simulink library "Lib_EMTAT"  (R2023b)
settings: Solver=VariableStepAuto  StartTime=0.0  StopTime=10.0  RelTol=1e-3
undefined symbols (not defined in the file or in its folder): MWS
libraries: simulink x31, $bdroot x1
(part 2 of 4)

== system Lib_EMTAT/Components/Power Flow/Battery ==
  note: Sign Convention:
      | i > 0 => discharging
      | i < 0 => charging
  note: Current Demand
  note: Depth of Discharge ( $\int i dt$ )
  note: Placeholder Power Loss Calculation (P = I^2*R)
  note: 1 = Discharging
      | 0 = Charging
  note: Depth of Charge/Discharge Calculation
  note: Voltage drop across resistance
  "I, A" : Inport
  "DoD, C" : Inport  Port=2
  A*s to Ah : Gain  Gain=1/3600
  Bus Creator : BusCreator  Inputs=6
  Charge Curve (1-D Lookup Table) : Lookup_n-D  NumberOfTableDimensions=1  BreakpointsForDimension1=It_vec  Table=Vcharge_vec  ExtrapMethod=Clip  UseLastTableValue=on  InternalRulePriority=Speed  RndMeth=Simplest
  Compare To Constant : simulink/Logic and Bit Operations/Compare To Constant  relop=>=  const=0  OutDataTypeStr=boolean
  Constant : Constant  Value=ESR
  Constant1 : Constant  Value=max(It_vec)
  Discharge Curve (1-D Lookup Table) : Lookup_n-D  NumberOfTableDimensions=1  BreakpointsForDimension1=It_vec  Table=Vdischarge_vec  ExtrapMethod=Clip  UseLastTableValue=on  InternalRulePriority=Speed  RndMeth=Simplest
  Divide4 : Product  Inputs=*/
  Product5 : Product
  Product8 : Product
  Saturation : Saturate  UpperLimit=100  LowerLimit=0
  Square : Math  Operator=square
  Subtract3 : Sum  Inputs=+-
  Subtract6 : Sum  Inputs=+-
  Switch : Switch  Criteria=u2 > Threshold  SaturateOnIntegerOverflow=off  InputSameDT=off
  to % : Gain  Gain=100
  "V, V" : Outport
  Outputs : Outport  Port=2
  "Ploss, W" : Outport  Port=3
  "I, C/s " : Outport  Port=4
  wires:
  [it] -> Bus Creator/6  "DoD_C"
  A*s to Ah/1 -> [it]
  "DoD, C"/1 -> A*s to Ah/1
  to %/1 -> Saturation/1
  Compare To Constant/1 -> [State], Bus Creator/5  "State"
  [i] -> Compare To Constant/1
  Product8/1 -> "Ploss, W"/1, Bus Creator/4  "Ploss_W"
  Square/1 -> Product8/2
  Constant/1 -> [R], Product8/1
  [i] -> Square/1  "i"
  [i] -> Bus Creator/3  "I_A"
  [SoC] -> Bus Creator/2  "SoC_%"
  Divide4/1 -> to %/1
  [Vout] -> Bus Creator/1  "V_V"
  Bus Creator/1 -> Outputs/1
  "I, A"/1 -> "I, C/s "/1, [i]
  Subtract6/1 -> Divide4/1
  [it] -> Subtract6/2
  Constant1/1 -> Subtract6/1, Divide4/2
  [it] -> Charge Curve (1-D Lookup Table)/1
  Subtract3/1 -> [Vout], "V, V"/1
  [R] -> Product5/1
  [i] -> Product5/2
  Product5/1 -> Subtract3/2
  Charge Curve (1-D Lookup Table)/1 -> Switch/3
  Saturation/1 -> [SoC]
  [State] -> Switch/2
  [it] -> Discharge Curve (1-D Lookup Table)/1
  Discharge Curve (1-D Lookup Table)/1 -> Switch/1
  Switch/1 -> Subtract3/1

== system Lib_EMTAT/Components/Power Flow/Cable ==
  note: Memory block used to break algebraic loop.
  "V_1, V" : Inport
  "I, A" : Inport  Port=2
  Fail? : Inport  Port=3
  "I(t-1), A" : Inport  Port=4
  Bus Creator : BusCreator  Inputs=7
  Constant : Constant  Value=R
  Divide{,1..3} (4 alike) : Product  Inputs=**
  Failure Determination : Subsystem
  Fix Zero Voltage Problem : Subsystem
  Open Circuit Failure - Current : Subsystem
  Open Circuit Failure - Voltage : Subsystem
  Square : Math  Operator=square
  Sum : Sum  Inputs=|-+
  "V_2, V" : Outport
  Outputs : Outport  Port=2
  "Ploss, W" : Outport  Port=3
  "I, A " : Outport  Port=4
  "I(t), A" : Outport  Port=5
  wires:
  [OCFail] -> Open Circuit Failure - Voltage/1(Failed?)
  Fix Zero Voltage Problem/1(Vout) -> Open Circuit Failure - Voltage/2(Vout)
  [OCFail] -> Open Circuit Failure - Current/1(Failed?)
  Open Circuit Failure - Current/1("Iin/Iout ") -> "I, A "/1, [Iin], Divide2/2, Divide3/1, Square/1
  "I, A"/1 -> "I(t), A"/1, Open Circuit Failure - Current/2(Iin/Iout)
  Fail?/1 -> Failure Determination/1(Fail?)
  Failure Determination/1(OCFail) -> [OCFail]
  "I(t-1), A"/1 -> Divide/1
  Divide/1 -> Sum/1
  "V_1, V"/1 -> Divide2/1, Sum/2, Fix Zero Voltage Problem/2(Vin), [Vin]
  Sum/1 -> Fix Zero Voltage Problem/1("Vout "), Divide3/2
  [Iin] -> Bus Creator/3  "I_A"
  [Vout] -> Bus Creator/5  "V_2_V"
  [Vin] -> Bus Creator/4  "V_1_V"
  Bus Creator/1 -> Outputs/1
  [R] -> Bus Creator/6  "R_ohm"
  Constant/1 -> Divide1/2, [R], Divide/2
  Square/1 -> Divide1/1
  Divide1/1 -> [Ploss], "Ploss, W"/1
  [Pin] -> Bus Creator/2  "P_1_W"
  [Pout] -> Bus Creator/1  "P_2_W"
  Divide2/1 -> [Pin]
  Divide3/1 -> [Pout]
  [Ploss] -> Bus Creator/7  "Ploss_W"
  Open Circuit Failure - Voltage/1("Vout ") -> "V_2, V"/1, [Vout]

== system Lib_EMTAT/Components/Power Flow/Current Distribution ==
  "I, A" : Inport
  "Idmd, A" : Inport  Port=2
  MATLAB Function : MATLAB Function  TreatAsAtomicUnit=on
  "Isplit, A" : Outport
  wires:
  "Idmd, A"/1 -> MATLAB Function/2(Idmd)
  MATLAB Function/1(Isplit) -> "Isplit, A"/1
  "I, A"/1 -> MATLAB Function/1(I)

== system Lib_EMTAT/Components/Power Flow/Current Junction ==
  I : Inport
  MATLAB Function : MATLAB Function  TreatAsAtomicUnit=on
  Isum : Outport
  wires:
  I/1 -> MATLAB Function/1(u)
  MATLAB Function/1(y) -> Isum/1

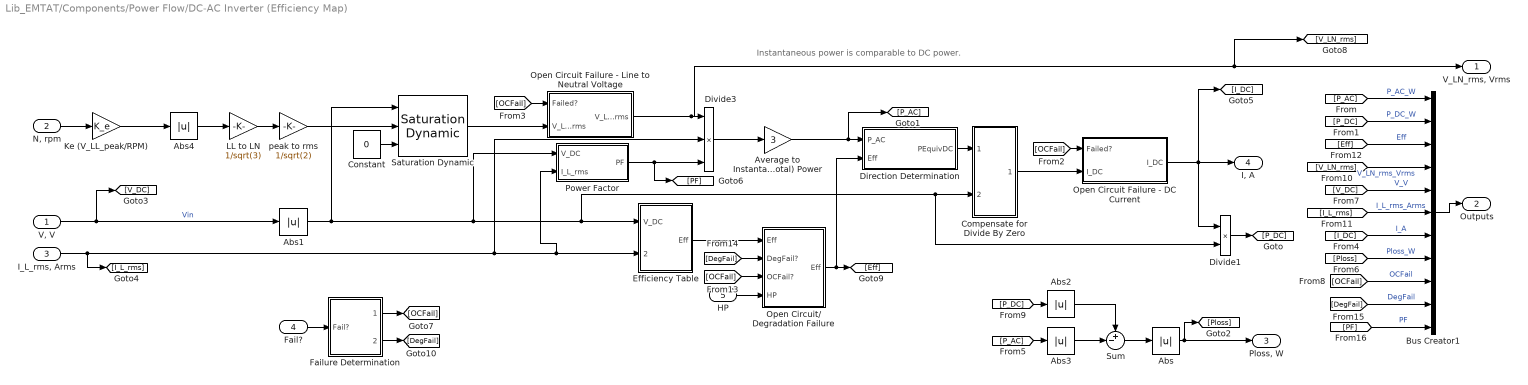
== system Lib_EMTAT/Components/Power Flow/DC-AC Inverter (Efficiency Map) ==
  note: Instantaneous power is comparable to DC power.
  "V, V" : Inport
  "N, rpm" : Inport  Port=2
  "I_L_rms, Arms" : Inport  Port=3
  Fail? : Inport  Port=4
  HP : Inport  Port=5
  Abs{,1..4} (5 alike) : Abs  SaturateOnIntegerOverflow=off
  Average to Instantaneous (Total) Power : Gain  Gain=3
  Bus Creator1 : BusCreator  Inputs=11
  Compensate for Divide By Zero : Subsystem
  Constant : Constant  Value=0
  Direction Determination : Subsystem
  Divide1 : Product  Inputs=**
  Divide3 : Product  Inputs=***
  Efficiency Table : Subsystem
  Failure Determination : Subsystem
  Ke (V_LL_peak/RPM) : Gain  Gain=K_e
  LL to LN : Gain  Gain=1/sqrt(3)
  Open Circuit Failure - DC Current : Subsystem
  Open Circuit Failure - Line to Neutral Voltage : Subsystem
  Open Circuit/ Degradation Failure : Subsystem
  Power Factor : Subsystem
  Saturation Dynamic : simulink/Discontinuities/Saturation Dynamic  OutMin=[]  OutMax=[]  OutDataTypeStr=Inherit: Same as second input  OutDataType=fixdt(1, 16)  OutScaling=2^-10  DoSatur=off
  Sum : Sum  Inputs=+-|
  peak to rms : Gain  Gain=1/sqrt(2)
  "V_LN_rms, Vrms" : Outport
  Outputs : Outport  Port=2
  "Ploss, W" : Outport  Port=3
  "I, A" : Outport  Port=4
  wires:
  peak to rms/1 -> Saturation Dynamic/2
  Constant/1 -> Saturation Dynamic/3
  Divide3/1 -> Average to Instantaneous (Total) Power/1
  Abs4/1 -> LL to LN/1
  Abs1/1 -> Power Factor/1(V_DC), Efficiency Table/1(V_DC), Compensate for Divide By Zero/2(V_DC), Divide1/2, Saturation Dynamic/1
  Divide1/1 -> [P_DC]
  Direction Determination/1(PEquivDC) -> Compensate for Divide By Zero/1(PEquivDC)
  Bus Creator1/1 -> Outputs/1
  [P_AC] -> Bus Creator1/1  "P_AC_W"
  [P_DC] -> Bus Creator1/2  "P_DC_W"
  "N, rpm"/1 -> Ke (V_LL_peak/RPM)/1
  Open Circuit/ Degradation Failure/1("Eff ") -> [Eff], Direction Determination/2(Eff)
  Open Circuit Failure - DC Current/1("I_DC ") -> Divide1/1, "I, A"/1, [I_DC]
  Average to Instantaneous (Total) Power/1 -> Direction Determination/1(P_AC), [P_AC]
  "V, V"/1 -> Abs1/1, [V_DC]  "Vin"
  Ke (V_LL_peak/RPM)/1 -> Abs4/1
  "I_L_rms, Arms"/1 -> Power Factor/2(I_L_rms), Efficiency Table/2(I_L_rms), Divide3/2, [I_L_rms]
  [V_LN_rms] -> Bus Creator1/4  "V_LN_rms_Vrms"
  [V_DC] -> Bus Creator1/5  "V_V"
  [I_DC] -> Bus Creator1/7  "I_A"
  [Ploss] -> Bus Creator1/8  "Ploss_W"
  [I_L_rms] -> Bus Creator1/6  "I_L_rms_Arms"
  [Eff] -> Bus Creator1/3  "Eff"
  LL to LN/1 -> peak to rms/1
  Compensate for Divide By Zero/1(I_DC) -> Open Circuit Failure - DC Current/2(I_DC)
  [OCFail] -> Open Circuit Failure - DC Current/1(Failed?)
  Saturation Dynamic/1 -> Open Circuit Failure - Line to Neutral Voltage/2(V_LN_rms)
  [OCFail] -> Open Circuit Failure - Line to Neutral Voltage/1(Failed?)
  Open Circuit Failure - Line to Neutral Voltage/1("V_LN_rms ") -> [V_LN_rms], "V_LN_rms, Vrms"/1, Divide3/1
  Efficiency Table/1(Eff) -> Open Circuit/ Degradation Failure/1(Eff)
  Failure Determination/2(DegFail) -> [DegFail]
  Failure Determination/1(OCFail) -> [OCFail]
  Fail?/1 -> Failure Determination/1(Fail?)
  HP/1 -> Open Circuit/ Degradation Failure/4(HP)
  [OCFail] -> Open Circuit/ Degradation Failure/3(OCFail?)
  [DegFail] -> Open Circuit/ Degradation Failure/2(DegFail?)
  Sum/1 -> Abs/1
  [P_DC] -> Abs2/1
  Abs3/1 -> Sum/2
  [P_AC] -> Abs3/1
  Abs2/1 -> Sum/1
  Abs/1 -> [Ploss], "Ploss, W"/1
  Power Factor/1(PF) -> [PF], Divide3/3
  [OCFail] -> Bus Creator1/9  "OCFail"
  [DegFail] -> Bus Creator1/10  "DegFail"
  [PF] -> Bus Creator1/11  "PF"

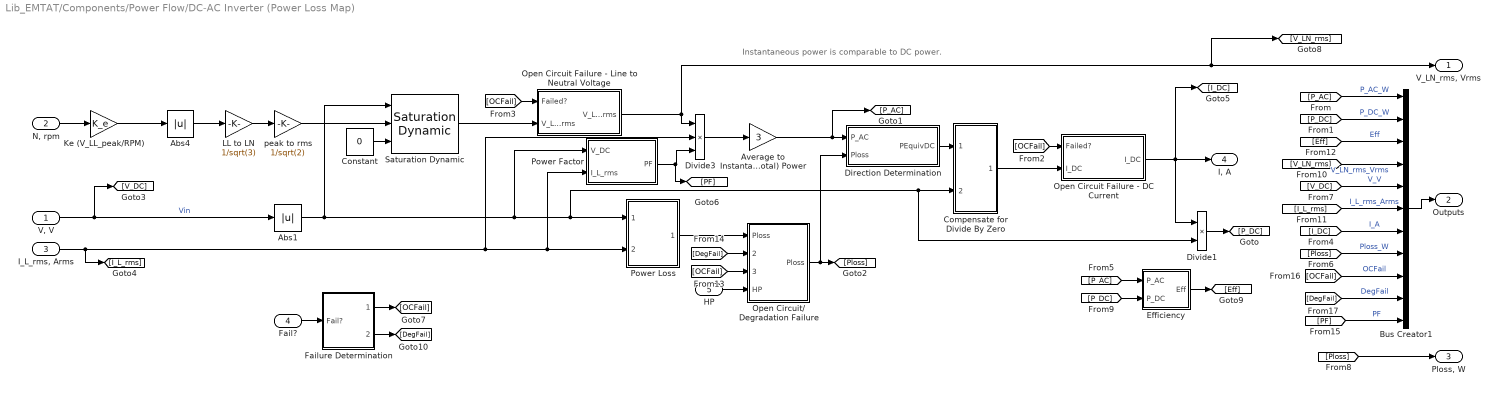
== system Lib_EMTAT/Components/Power Flow/DC-AC Inverter (Power Loss Map) ==
  note: Instantaneous power is comparable to DC power.
  "V, V" : Inport
  "N, rpm" : Inport  Port=2
  "I_L_rms, Arms" : Inport  Port=3
  Fail? : Inport  Port=4
  HP : Inport  Port=5
  Abs1 : Abs  SaturateOnIntegerOverflow=off
  Abs4 : Abs  SaturateOnIntegerOverflow=off
  Average to Instantaneous (Total) Power : Gain  Gain=3
  Bus Creator1 : BusCreator  Inputs=11
  Compensate for Divide By Zero : Subsystem
  Constant : Constant  Value=0
  Direction Determination : Subsystem
  Divide1 : Product  Inputs=**
  Divide3 : Product  Inputs=***
  Efficiency : Subsystem
  Failure Determination : Subsystem
  Ke (V_LL_peak/RPM) : Gain  Gain=K_e
  LL to LN : Gain  Gain=1/sqrt(3)
  Open Circuit Failure - DC Current : Subsystem
  Open Circuit Failure - Line to Neutral Voltage : Subsystem
  Open Circuit/ Degradation Failure : Subsystem
  Power Factor : Subsystem
  Power Loss : Subsystem
  Saturation Dynamic : simulink/Discontinuities/Saturation Dynamic  OutMin=[]  OutMax=[]  OutDataTypeStr=Inherit: Same as second input  OutDataType=fixdt(1, 16)  OutScaling=2^-10  DoSatur=off
  peak to rms : Gain  Gain=1/sqrt(2)
  "V_LN_rms, Vrms" : Outport
  Outputs : Outport  Port=2
  "Ploss, W" : Outport  Port=3
  "I, A" : Outport  Port=4
  wires:
  [DegFail] -> Open Circuit/ Degradation Failure/2(DegFail?)
  [OCFail] -> Open Circuit/ Degradation Failure/3(OCFail?)
  HP/1 -> Open Circuit/ Degradation Failure/4(HP)
  Fail?/1 -> Failure Determination/1(Fail?)
  Failure Determination/1(OCFail) -> [OCFail]
  Failure Determination/2(DegFail) -> [DegFail]
  Power Loss/1(Ploss) -> Open Circuit/ Degradation Failure/1(Ploss)
  Open Circuit Failure - Line to Neutral Voltage/1("V_LN_rms ") -> Divide3/1, "V_LN_rms, Vrms"/1, [V_LN_rms]
  [OCFail] -> Open Circuit Failure - Line to Neutral Voltage/1(Failed?)
  Saturation Dynamic/1 -> Open Circuit Failure - Line to Neutral Voltage/2(V_LN_rms)
  [OCFail] -> Open Circuit Failure - DC Current/1(Failed?)
  Compensate for Divide By Zero/1(I_DC) -> Open Circuit Failure - DC Current/2(I_DC)
  LL to LN/1 -> peak to rms/1
  [Eff] -> Bus Creator1/3  "Eff"
  Efficiency/1(Eff) -> [Eff]
  [P_AC] -> Efficiency/1(P_AC)
  [P_DC] -> Efficiency/2(P_DC)
  [I_L_rms] -> Bus Creator1/6  "I_L_rms_Arms"
  [Ploss] -> Bus Creator1/8  "Ploss_W"
  [I_DC] -> Bus Creator1/7  "I_A"
  [V_DC] -> Bus Creator1/5  "V_V"
  [V_LN_rms] -> Bus Creator1/4  "V_LN_rms_Vrms"
  "I_L_rms, Arms"/1 -> [I_L_rms], Divide3/2, Power Factor/2(I_L_rms), Power Loss/2(I_L_rms)
  [Ploss] -> "Ploss, W"/1
  Ke (V_LL_peak/RPM)/1 -> Abs4/1
  "V, V"/1 -> [V_DC], Abs1/1  "Vin"
  Average to Instantaneous (Total) Power/1 -> [P_AC], Direction Determination/1(P_AC)
  Open Circuit Failure - DC Current/1("I_DC ") -> [I_DC], "I, A"/1, Divide1/1
  Open Circuit/ Degradation Failure/1("Ploss ") -> [Ploss], Direction Determination/2(Ploss)
  "N, rpm"/1 -> Ke (V_LL_peak/RPM)/1
  [P_DC] -> Bus Creator1/2  "P_DC_W"
  [P_AC] -> Bus Creator1/1  "P_AC_W"
  Bus Creator1/1 -> Outputs/1
  Direction Determination/1(PEquivDC) -> Compensate for Divide By Zero/1(PEquivDC)
  Divide1/1 -> [P_DC]
  Abs1/1 -> Saturation Dynamic/1, Power Factor/1(V_DC), Divide1/2, Compensate for Divide By Zero/2(V_DC), Power Loss/1(V_DC)
  Abs4/1 -> LL to LN/1
  Divide3/1 -> Average to Instantaneous (Total) Power/1
  Constant/1 -> Saturation Dynamic/3
  peak to rms/1 -> Saturation Dynamic/2
  Power Factor/1(PF) -> [PF], Divide3/3
  [OCFail] -> Bus Creator1/9  "OCFail"
  [DegFail] -> Bus Creator1/10  "DegFail"
  [PF] -> Bus Creator1/11  "PF"

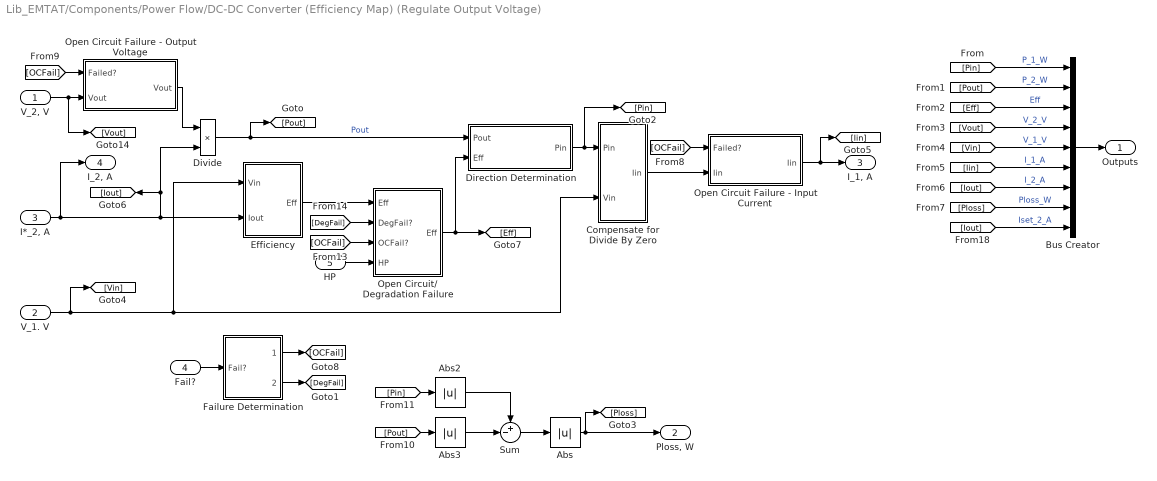
== system Lib_EMTAT/Components/Power Flow/DC-DC Converter (Efficiency Map) (Regulate Output Voltage) ==
  "V_2, V" : Inport
  V_1. V : Inport  Port=2
  "I*_2, A" : Inport  Port=3
  Fail? : Inport  Port=4
  HP : Inport  Port=5
  Abs : Abs  SaturateOnIntegerOverflow=off
  Abs2 : Abs  SaturateOnIntegerOverflow=off
  Abs3 : Abs  SaturateOnIntegerOverflow=off
  Bus Creator : BusCreator  Inputs=9
  Compensate for Divide By Zero : Subsystem
  Direction Determination : Subsystem
  Divide : Product  Inputs=**
  Efficiency : Subsystem
  Failure Determination : Subsystem
  Open Circuit Failure - Input Current : Subsystem
  Open Circuit Failure - Output Voltage : Subsystem
  Open Circuit/ Degradation Failure : Subsystem
  Sum : Sum  Inputs=+-|
  Outputs : Outport
  "Ploss, W" : Outport  Port=2
  "I_1, A" : Outport  Port=3
  "I_2, A" : Outport  Port=4
  wires:
  [Iout] -> Bus Creator/9  "Iset_2_A"
  Fail?/1 -> Failure Determination/1(Fail?)
  Failure Determination/1(OCFail) -> [OCFail]
  Failure Determination/2(DegFail) -> [DegFail]
  Efficiency/1(Eff) -> Open Circuit/ Degradation Failure/1(Eff)
  HP/1 -> Open Circuit/ Degradation Failure/4(HP)
  [DegFail] -> Open Circuit/ Degradation Failure/2(DegFail?)
  [OCFail] -> Open Circuit/ Degradation Failure/3(OCFail?)
  [OCFail] -> Open Circuit Failure - Output Voltage/1(Failed?)
  Open Circuit Failure - Output Voltage/1("Vout   ") -> Divide/1
  [OCFail] -> Open Circuit Failure - Input Current/1(Failed?)
  Compensate for Divide By Zero/1(Iin) -> Open Circuit Failure - Input Current/2(Iin)
  "V_2, V"/1 -> Open Circuit Failure - Output Voltage/2(Vout), [Vout]
  V_1. V/1 -> [Vin], Compensate for Divide By Zero/2(Vin), Efficiency/1(Vin)
  Open Circuit Failure - Input Current/1("Iin  ") -> "I_1, A"/1, [Iin]
  Open Circuit/ Degradation Failure/1("Eff ") -> Direction Determination/2(Eff), [Eff]
  Divide/1 -> Direction Determination/1(Pout), [Pout]  "Pout"
  Bus Creator/1 -> Outputs/1
  Direction Determination/1(Pin) -> [Pin], Compensate for Divide By Zero/1(Pin)
  [Pin] -> Bus Creator/1  "P_1_W"
  [Pout] -> Bus Creator/2  "P_2_W"
  [Eff] -> Bus Creator/3  "Eff"
  [Vout] -> Bus Creator/4  "V_2_V"
  [Vin] -> Bus Creator/5  "V_1_V"
  [Iin] -> Bus Creator/6  "I_1_A"
  "I*_2, A"/1 -> "I_2, A"/1, Efficiency/2(Iout), [Iout], Divide/2
  [Iout] -> Bus Creator/7  "I_2_A"
  [Pout] -> Abs3/1
  Abs3/1 -> Sum/2
  [Pin] -> Abs2/1
  Sum/1 -> Abs/1
  Abs2/1 -> Sum/1
  Abs/1 -> "Ploss, W"/1, [Ploss]
  [Ploss] -> Bus Creator/8  "Ploss_W"

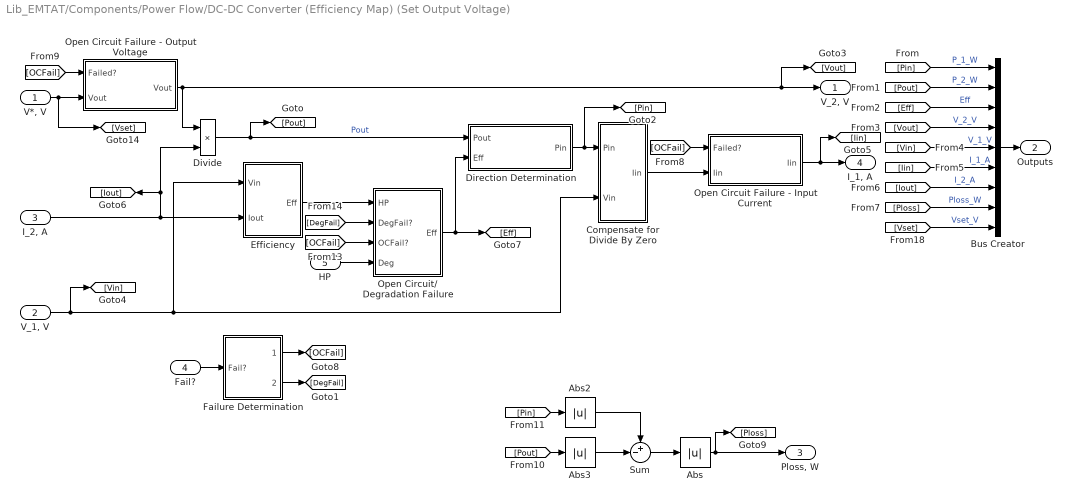
== system Lib_EMTAT/Components/Power Flow/DC-DC Converter (Efficiency Map) (Set Output Voltage) ==
  "V*, V" : Inport
  "V_1, V" : Inport  Port=2
  "I_2, A" : Inport  Port=3
  Fail? : Inport  Port=4
  HP : Inport  Port=5
  Abs : Abs  SaturateOnIntegerOverflow=off
  Abs2 : Abs  SaturateOnIntegerOverflow=off
  Abs3 : Abs  SaturateOnIntegerOverflow=off
  Bus Creator : BusCreator  Inputs=9
  Compensate for Divide By Zero : Subsystem
  Direction Determination : Subsystem
  Divide : Product  Inputs=**
  Efficiency : Subsystem
  Failure Determination : Subsystem
  Open Circuit Failure - Input Current : Subsystem
  Open Circuit Failure - Output Voltage : Subsystem
  Open Circuit/ Degradation Failure : Subsystem
  Sum : Sum  Inputs=+-|
  "V_2, V" : Outport
  Outputs : Outport  Port=2
  "Ploss, W" : Outport  Port=3
  "I_1, A" : Outport  Port=4
  wires:
  [Ploss] -> Bus Creator/8  "Ploss_W"
  [Iout] -> Bus Creator/7  "I_2_A"
  "I_2, A"/1 -> Divide/2, [Iout], Efficiency/2(Iout)
  [Iin] -> Bus Creator/6  "I_1_A"
  [Vin] -> Bus Creator/5  "V_1_V"
  [Vout] -> Bus Creator/4  "V_2_V"
  [Eff] -> Bus Creator/3  "Eff"
  [Pout] -> Bus Creator/2  "P_2_W"
  [Pin] -> Bus Creator/1  "P_1_W"
  Direction Determination/1(Pin) -> Compensate for Divide By Zero/1(Pin), [Pin]
  Bus Creator/1 -> Outputs/1
  Divide/1 -> Direction Determination/1(Pout), [Pout]  "Pout"
  Open Circuit/ Degradation Failure/1("Eff ") -> Direction Determination/2(Eff), [Eff]
  Open Circuit Failure - Input Current/1("Iin  ") -> "I_1, A"/1, [Iin]
  "V_1, V"/1 -> Efficiency/1(Vin), Compensate for Divide By Zero/2(Vin), [Vin]
  "V*, V"/1 -> [Vset], Open Circuit Failure - Output Voltage/2(Vout)
  Compensate for Divide By Zero/1(Iin) -> Open Circuit Failure - Input Current/2(Iin)
  [OCFail] -> Open Circuit Failure - Input Current/1(Failed?)
  Open Circuit Failure - Output Voltage/1("Vout   ") -> [Vout], "V_2, V"/1, Divide/1
  [OCFail] -> Open Circuit Failure - Output Voltage/1(Failed?)
  [OCFail] -> Open Circuit/ Degradation Failure/3(OCFail?)
  [DegFail] -> Open Circuit/ Degradation Failure/2(DegFail?)
  HP/1 -> Open Circuit/ Degradation Failure/4(Deg)
  Efficiency/1(Eff) -> Open Circuit/ Degradation Failure/1(HP)
  Failure Determination/2(DegFail) -> [DegFail]
  Failure Determination/1(OCFail) -> [OCFail]
  Fail?/1 -> Failure Determination/1(Fail?)
  [Vset] -> Bus Creator/9  "Vset_V"
  Abs/1 -> "Ploss, W"/1, [Ploss]
  Abs3/1 -> Sum/2
  [Pout] -> Abs3/1
  Sum/1 -> Abs/1
  Abs2/1 -> Sum/1
  [Pin] -> Abs2/1

== system Lib_EMTAT/Components/Power Flow/DC-DC Converter (Power Loss Map) (Regulate Output Voltage) ==
  "V_2, V" : Inport
  V_1. V : Inport  Port=2
  "I*_2, A" : Inport  Port=3
  Fail? : Inport  Port=4
  HP : Inport  Port=5
  Bus Creator : BusCreator  Inputs=13
  Compensate for Divide By Zero : Subsystem
  Direction Determination : Subsystem
  Divide : Product  Inputs=**
  Efficiency : Subsystem
  Failure Determination : Subsystem
  Open Circuit Failure - Input Current : Subsystem
  Open Circuit Failure - Output Voltage : Subsystem
  Open Circuit/ Degradation Failure : Subsystem
  Power Loss : Subsystem
  Outputs : Outport
  "Ploss, W" : Outport  Port=2
  "I_1, A" : Outport  Port=3
  "I_2, A" : Outport  Port=4
  wires:
  [Ploss] -> Bus Creator/8  "Ploss_W"
  [Iout] -> Bus Creator/7  "I_2_A"
  "I*_2, A"/1 -> Divide/2, [Iout], Power Loss/2(Iout), "I_2, A"/1
  [Iin] -> Bus Creator/6  "I_1_A"
  [Vin] -> Bus Creator/5  "V_1_V"
  [Vout] -> Bus Creator/4  "V_2_V"
  [Eff] -> Bus Creator/3  "Eff"
  [Pout] -> Bus Creator/2  "P_2_W"
  [Pin] -> Bus Creator/1  "P_1_W"
  Direction Determination/1(Pin) -> Compensate for Divide By Zero/1(Pin), [Pin]
  Bus Creator/1 -> Outputs/1
  Divide/1 -> Direction Determination/1(Pout), [Pout]  "Pout"
  Open Circuit/ Degradation Failure/1("Ploss ") -> "Ploss, W"/1, Direction Determination/2(Ploss), [Ploss]
  Open Circuit Failure - Input Current/1("Iin  ") -> [Iin], "I_1, A"/1
  V_1. V/1 -> Power Loss/1(Vin), Compensate for Divide By Zero/2(Vin), [Vin]
  "V_2, V"/1 -> [Vout], Open Circuit Failure - Output Voltage/2(Vout)
  [Pout] -> Efficiency/1(Pout)
  [Pin] -> Efficiency/2(Pin)
  Efficiency/1(Eff) -> [Eff]
  Compensate for Divide By Zero/1(Iin) -> Open Circuit Failure - Input Current/2(Iin)
  [OCFail] -> Open Circuit Failure - Input Current/1(Failed?)
  Open Circuit Failure - Output Voltage/1("Vout   ") -> Divide/1
  [OCFail] -> Open Circuit Failure - Output Voltage/1(Failed?)
  [OCFail] -> Open Circuit/ Degradation Failure/3(OCFail?)
  [DegFail] -> Open Circuit/ Degradation Failure/2(DegFail?)
  HP/1 -> Open Circuit/ Degradation Failure/4(HP)
  Power Loss/1(Ploss) -> Open Circuit/ Degradation Failure/1(Ploss)
  Failure Determination/2(DegFail) -> [DegFail]
  Failure Determination/1(OCFail) -> [OCFail]
  Fail?/1 -> Failure Determination/1(Fail?)
  [Iout] -> Bus Creator/9  "Iset_2_A"

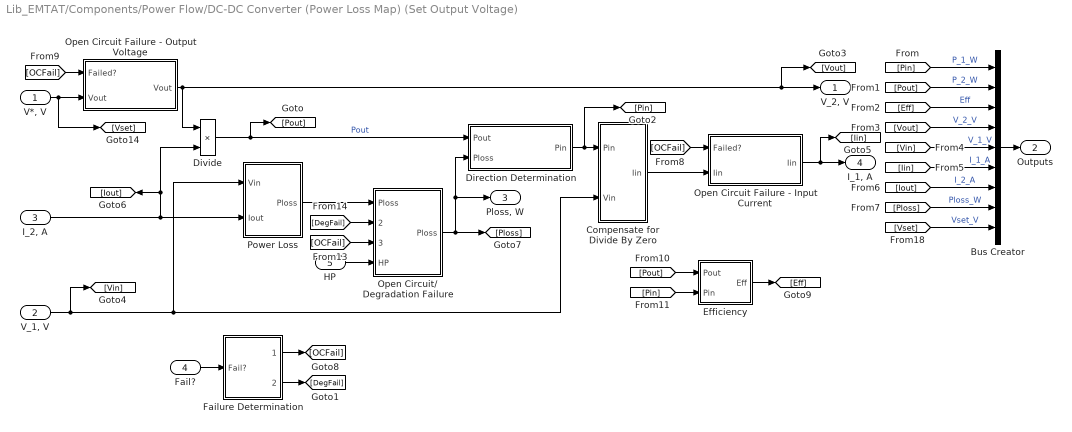
== system Lib_EMTAT/Components/Power Flow/DC-DC Converter (Power Loss Map) (Set Output Voltage) ==
  "V*, V" : Inport
  "V_1, V" : Inport  Port=2
  "I_2, A" : Inport  Port=3
  Fail? : Inport  Port=4
  HP : Inport  Port=5
  Bus Creator : BusCreator  Inputs=9
  Compensate for Divide By Zero : Subsystem
  Direction Determination : Subsystem
  Divide : Product  Inputs=**
  Efficiency : Subsystem
  Failure Determination : Subsystem
  Open Circuit Failure - Input Current : Subsystem
  Open Circuit Failure - Output Voltage : Subsystem
  Open Circuit/ Degradation Failure : Subsystem
  Power Loss : Subsystem
  "V_2, V" : Outport
  Outputs : Outport  Port=2
  "Ploss, W" : Outport  Port=3
  "I_1, A" : Outport  Port=4
  wires:
  [Vset] -> Bus Creator/9  "Vset_V"
  Fail?/1 -> Failure Determination/1(Fail?)
  Failure Determination/1(OCFail) -> [OCFail]
  Failure Determination/2(DegFail) -> [DegFail]
  Power Loss/1(Ploss) -> Open Circuit/ Degradation Failure/1(Ploss)
  HP/1 -> Open Circuit/ Degradation Failure/4(HP)
  [DegFail] -> Open Circuit/ Degradation Failure/2(DegFail?)
  [OCFail] -> Open Circuit/ Degradation Failure/3(OCFail?)
  [OCFail] -> Open Circuit Failure - Output Voltage/1(Failed?)
  Open Circuit Failure - Output Voltage/1("Vout   ") -> Divide/1, "V_2, V"/1, [Vout]
  [OCFail] -> Open Circuit Failure - Input Current/1(Failed?)
  Compensate for Divide By Zero/1(Iin) -> Open Circuit Failure - Input Current/2(Iin)
  Efficiency/1(Eff) -> [Eff]
  [Pin] -> Efficiency/2(Pin)
  [Pout] -> Efficiency/1(Pout)
  "V*, V"/1 -> Open Circuit Failure - Output Voltage/2(Vout), [Vset]
  "V_1, V"/1 -> [Vin], Compensate for Divide By Zero/2(Vin), Power Loss/1(Vin)
  Open Circuit Failure - Input Current/1("Iin  ") -> [Iin], "I_1, A"/1
  Open Circuit/ Degradation Failure/1("Ploss ") -> [Ploss], Direction Determination/2(Ploss), "Ploss, W"/1
  Divide/1 -> [Pout], Direction Determination/1(Pout)  "Pout"
  Bus Creator/1 -> Outputs/1
  Direction Determination/1(Pin) -> [Pin], Compensate for Divide By Zero/1(Pin)
  [Pin] -> Bus Creator/1  "P_1_W"
  [Pout] -> Bus Creator/2  "P_2_W"
  [Eff] -> Bus Creator/3  "Eff"
  [Vout] -> Bus Creator/4  "V_2_V"
  [Vin] -> Bus Creator/5  "V_1_V"
  [Iin] -> Bus Creator/6  "I_1_A"
  "I_2, A"/1 -> Power Loss/2(Iout), [Iout], Divide/2
  [Iout] -> Bus Creator/7  "I_2_A"
  [Ploss] -> Bus Creator/8  "Ploss_W"

== system Lib_EMTAT/Components/Power Flow/Electrical Bus ==
  "I, A" : Inport
  "V, V" : Inport  Port=2
  "Capacitance, F" : Constant  Value=C
  Divide : Product  Inputs=*/
  MATLAB Function : MATLAB Function  TreatAsAtomicUnit=on
  "V, V " : Outport
  "Vdot, V/sec" : Outport  Port=2
  wires:
  MATLAB Function/1(y) -> Divide/1
  "Capacitance, F"/1 -> Divide/2
  Divide/1 -> "Vdot, V/sec"/1
  "V, V"/1 -> "V, V "/1
  "I, A"/1 -> MATLAB Function/1(u)

== system Lib_EMTAT/Components/Power Flow/Mechanical Shaft ==
  note: Units
      | J : lb-ft-s^2
      | B : lb-ft-s
  "T, lbf-ft" : Inport
  Fail? : Inport  Port=2
  "N, rpm" : Inport  Port=3
  Abs : Abs  SaturateOnIntegerOverflow=off
  Bus Creator : BusCreator  Inputs=5
  Divide : Product  Inputs=*/
  Divide1 : Product  Inputs=**
  Failure Determination : Subsystem
  Inertia (slug-ft^2 or lbf-ft-s^2) : Constant  Value=J
  RPM to rad/s : Gain  Gain=(2*pi)/60
  Shaft Break Failure : Subsystem
  Sum : Sum  Inputs=|+-
  "Viscous Damping Coefficient, lbf-ft-s" : Gain  Gain=B
  lbf-ft to N-m : Gain  Gain=1.355818
  rad/s^2 to RPM/s : Gain  Gain=60/(2*pi)
  Outputs : Outport
  "Ploss, W" : Outport  Port=2
  "Ndot, rpm/sec" : Outport  Port=3
  wires:
  Shaft Break Failure/1("T ") -> Sum/1
  [SBFail] -> Bus Creator/5  "SBFail"
  RPM to rad/s/1 -> Divide1/2, "Viscous Damping Coefficient, lbf-ft-s"/1
  [SBFail] -> Shaft Break Failure/1(Failed?)
  Fail?/1 -> Failure Determination/1(Fail?)
  Failure Determination/1(SBFail) -> [SBFail]
  "N, rpm"/1 -> RPM to rad/s/1, [N]
  [Ndot] -> Bus Creator/3  "Ndot_rpm/sec"
  Inertia (slug-ft^2 or lbf-ft-s^2)/1 -> Divide/2
  Bus Creator/1 -> Outputs/1
  rad/s^2 to RPM/s/1 -> [Ndot], "Ndot, rpm/sec"/1
  Divide/1 -> rad/s^2 to RPM/s/1
  [Tnet] -> Bus Creator/1  "Tnet_lbf-ft"
  [N] -> Bus Creator/2  "N_rpm"
  [Ploss] -> Bus Creator/4  "Ploss_W"
  Abs/1 -> "Ploss, W"/1, [Ploss]
  Sum/1 -> [Tnet], Divide/1
  "Viscous Damping Coefficient, lbf-ft-s"/1 -> Sum/2, lbf-ft to N-m/1
  lbf-ft to N-m/1 -> Divide1/1
  "T, lbf-ft"/1 -> Shaft Break Failure/2(T)
  Divide1/1 -> Abs/1

== system Lib_EMTAT/Components/Power Flow/Power Supply (Set Voltage) ==
  "V*, V" : Inport
  "I, A" : Inport  Port=2
  Bus Creator : BusCreator  Inputs=3
  Divide : Product  Inputs=**
  MATLAB Function : MATLAB Function  TreatAsAtomicUnit=on
  Outputs : Outport
  "V, V" : Outport  Port=2
  wires:
  [Pdmd] -> Bus Creator/3  "P_W"
  [Idmdsum] -> Bus Creator/2  "Isum_A"
  [Vout] -> Bus Creator/1  "V_V"
  Divide/1 -> [Pdmd]
  Bus Creator/1 -> Outputs/1
  "V*, V"/1 -> "V, V"/1, Divide/1, [Vout]
  MATLAB Function/1(y) -> [Idmdsum], Divide/2  "Isum"
  "I, A"/1 -> MATLAB Function/1(u)

== system Lib_EMTAT/Components/Power Flow/Resistive Load Bank ==
  "V, V" : Inport
  "P*, W " : Inport  Port=2
  Fail? : Inport  Port=3
  Abs1 : Abs  SaturateOnIntegerOverflow=off
  Bus Creator : BusCreator  Inputs=5
  Divide2 : Product  Inputs=**
  Failure Determination : Subsystem
  Fix Divide By Zero. : Subsystem
  Fix Divide By Zero.1 : Subsystem
  Open Circuit Failure - Line to Neutral Voltage : Subsystem
  Square : Math  Operator=square
  Outputs : Outport
  "Ploss, W" : Outport  Port=2
  "I, A" : Outport  Port=3
  wires:
  Fix Divide By Zero.1/1(I) -> Open Circuit Failure - Line to Neutral Voltage/2(I)
  [OCFail] -> Open Circuit Failure - Line to Neutral Voltage/1(Failed?)
  Fail?/1 -> Failure Determination/1(Fail?)
  Failure Determination/1(OCFail) -> [OCFail]
  Abs1/1 -> Fix Divide By Zero./2(abs(Pset))
  Fix Divide By Zero./1(R) -> [R], Divide2/2
  Bus Creator/1 -> Outputs/1
  Square/1 -> Divide2/1, Fix Divide By Zero./1(I^2)
  "P*, W "/1 -> [Pset], Abs1/1, Fix Divide By Zero.1/2(Pset)  "Pset"
  "V, V"/1 -> [V], Fix Divide By Zero.1/1(V)  "V"
  Divide2/1 -> [Ploss], "Ploss, W"/1
  [V] -> Bus Creator/1  "V_V"
  [I] -> Bus Creator/2  "I_A"
  [Pset] -> Bus Creator/3  "Pset_W"
  [R] -> Bus Creator/4  "R_ohm"
  [Ploss] -> Bus Creator/5  "Ploss_W"
  Open Circuit Failure - Line to Neutral Voltage/1("I ") -> Square/1, [I], "I, A"/1

== system Lib_EMTAT/Components/Power Flow/Supercapacitor ==
  note: Explanation for Convention Correction:
      | If Iout is positive, discharge the capacitor. This is because a positive current demand from a sink block means that the sink block needs current.
      | If Iout is negative, charge the capacitor. This is because a negative current demand from a sink block means that the sink block is giving current.
  "I, A " : Inport
  "V, V" : Inport  Port=2
  "I(t-1), A" : Inport  Port=3
  Bus Creator : BusCreator  Inputs=5
  Constant : Constant  Value=ESR
  Convention Correction : Gain  Gain=-1
  Divide : Product  Inputs=**
  Divide1 : Product  Inputs=**
  Gain : Gain  Gain=1/C
  SOC : Subsystem
  Saturation : Saturate  UpperLimit=inf  LowerLimit=0
  Square1 : Math  Operator=square
  Sum : Sum  Inputs=|-+
  "Voltage, V to Energy, Wh" : Subsystem
  Warnings : Subsystem
  "Vout, V" : Outport
  Outputs : Outport  Port=2
  "Ploss, W" : Outport  Port=3
  "Vdot, V/sec" : Outport  Port=4
  "I(t), A" : Outport  Port=5
  wires:
  Saturation/1 -> "Voltage, V to Energy, Wh"/1(V), "Vout, V"/1, [Vout]
  "I(t-1), A"/1 -> Convention Correction/1, Divide/1
  "V, V"/1 -> Sum/2
  Divide/1 -> Sum/1
  Constant/1 -> Divide/2, Divide1/2
  Sum/1 -> Saturation/1
  [SOC] -> Warnings/1(SOC)
  "Voltage, V to Energy, Wh"/1(E) -> [Energy], SOC/1(Energy (W-h))
  "I, A "/1 -> [Iout], "I(t), A"/1
  SOC/1(SOC) -> [SOC]
  [SOC] -> Bus Creator/4  "SoC_perc"
  Divide1/1 -> [Ploss], "Ploss, W"/1
  [Ploss] -> Bus Creator/5  "Ploss_W"
  Square1/1 -> Divide1/1
  Bus Creator/1 -> Outputs/1
  [Vout] -> Bus Creator/3  "Vout_V"
  [Iout] -> Bus Creator/2  "I_A"
  [Energy] -> Bus Creator/1  "E_Wh"
  Gain/1 -> "Vdot, V/sec"/1  "Vdot"
  Convention Correction/1 -> Gain/1, Square1/1

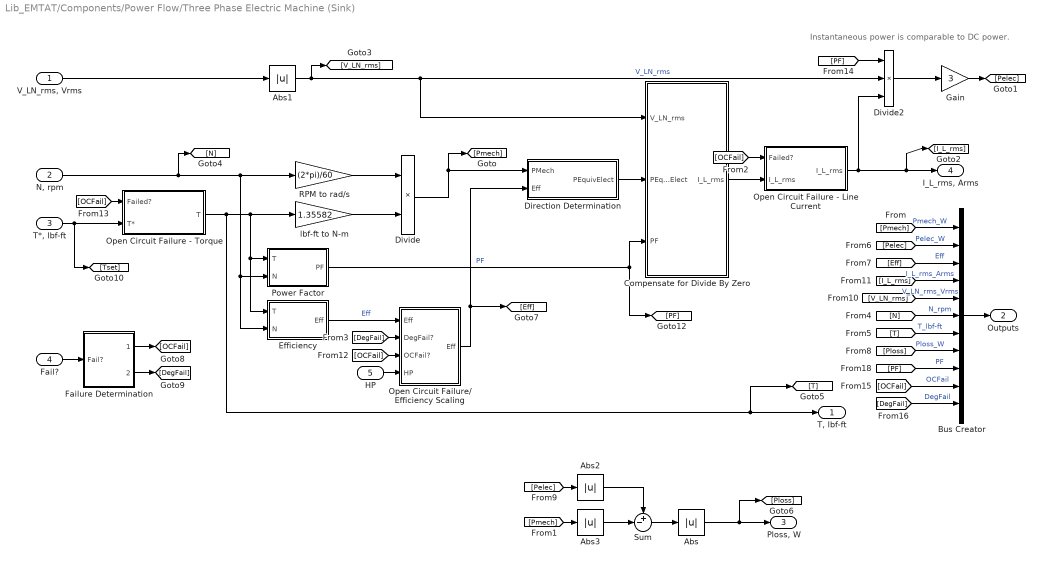
== system Lib_EMTAT/Components/Power Flow/Three Phase Electric Machine (Sink) ==
  note: Instantaneous power is comparable to DC power.
  "V_LN_rms, Vrms" : Inport
  "N, rpm" : Inport  Port=2
  "T*, lbf-ft" : Inport  Port=3
  Fail? : Inport  Port=4
  HP : Inport  Port=5
  Abs{,1..3} (4 alike) : Abs  SaturateOnIntegerOverflow=off
  Bus Creator : BusCreator  Inputs=11
  Compensate for Divide By Zero : Subsystem
  Direction Determination : Subsystem
  Divide : Product  Inputs=**
  Divide2 : Product  Inputs=***
  Efficiency : Subsystem
  Failure Determination : Subsystem
  Gain : Gain  Gain=3
  Open Circuit Failure - Line Current : Subsystem
  Open Circuit Failure - Torque : Subsystem
  Open Circuit Failure/ Efficiency Scaling : Subsystem
  Power Factor : Subsystem
  RPM to rad/s : Gain  Gain=(2*pi)/60
  Sum : Sum  Inputs=+-|
  lbf-ft to N-m : Gain  Gain=1.35582
  "T, lbf-ft" : Outport
  Outputs : Outport  Port=2
  "Ploss, W" : Outport  Port=3
  "I_L_rms, Arms" : Outport  Port=4
  wires:
  [DegFail] -> Bus Creator/11  "DegFail"
  [OCFail] -> Bus Creator/10  "OCFail"
  "T*, lbf-ft"/1 -> [Tset], Open Circuit Failure - Torque/2(T*)
  [OCFail] -> Open Circuit Failure - Torque/1(Failed?)
  [OCFail] -> Open Circuit Failure/ Efficiency Scaling/3(OCFail?)
  Fail?/1 -> Failure Determination/1(Fail?)
  HP/1 -> Open Circuit Failure/ Efficiency Scaling/4(HP)
  [DegFail] -> Open Circuit Failure/ Efficiency Scaling/2(DegFail?)
  Open Circuit Failure/ Efficiency Scaling/1("Eff ") -> [Eff], Direction Determination/2(Eff)
  Failure Determination/2(DegFail) -> [DegFail]
  Failure Determination/1(OCFail) -> [OCFail]
  [OCFail] -> Open Circuit Failure - Line Current/1(Failed?)
  Compensate for Divide By Zero/1(I_L_rms) -> Open Circuit Failure - Line Current/2(I_L_rms)
  Open Circuit Failure - Line Current/1("I_L_rms ") -> Divide2/3, "I_L_rms, Arms"/1, [I_L_rms]
  [N] -> Bus Creator/6  "N_rpm"
  [I_L_rms] -> Bus Creator/4  "I_L_rms_Arms"
  [V_LN_rms] -> Bus Creator/5  "V_LN_rms_Vrms"
  Abs1/1 -> [V_LN_rms], Compensate for Divide By Zero/1(V_LN_rms), Divide2/2  "V_LN_rms"
  Abs3/1 -> Sum/2
  [Pmech] -> Abs3/1
  Abs2/1 -> Sum/1
  [Pelec] -> Abs2/1
  Bus Creator/1 -> Outputs/1
  Efficiency/1(Eff) -> Open Circuit Failure/ Efficiency Scaling/1(Eff)  "Eff"
  "V_LN_rms, Vrms"/1 -> Abs1/1
  lbf-ft to N-m/1 -> Divide/2
  RPM to rad/s/1 -> Divide/1
  Open Circuit Failure - Torque/1("T  ") -> Power Factor/1(T), Efficiency/1(T), lbf-ft to N-m/1, "T, lbf-ft"/1, [T]
  Divide/1 -> [Pmech], Direction Determination/1(PMech)
  [Pmech] -> Bus Creator/1  "Pmech_W"
  Divide2/1 -> Gain/1
  [T] -> Bus Creator/7  "T_lbf-ft"
  [Eff] -> Bus Creator/3  "Eff"
  [Ploss] -> Bus Creator/8  "Ploss_W"
  Sum/1 -> Abs/1
  [Pelec] -> Bus Creator/2  "Pelec_W"
  Abs/1 -> [Ploss], "Ploss, W"/1
  Direction Determination/1(PEquivElect) -> Compensate for Divide By Zero/2(PEquivElect)
  "N, rpm"/1 -> Efficiency/2(N), Power Factor/2(N), RPM to rad/s/1, [N]
  Gain/1 -> [Pelec]
  Power Factor/1(PF) -> Compensate for Divide By Zero/3(PF), [PF]  "PF"
  [PF] -> Bus Creator/9  "PF"
  [PF] -> Divide2/1

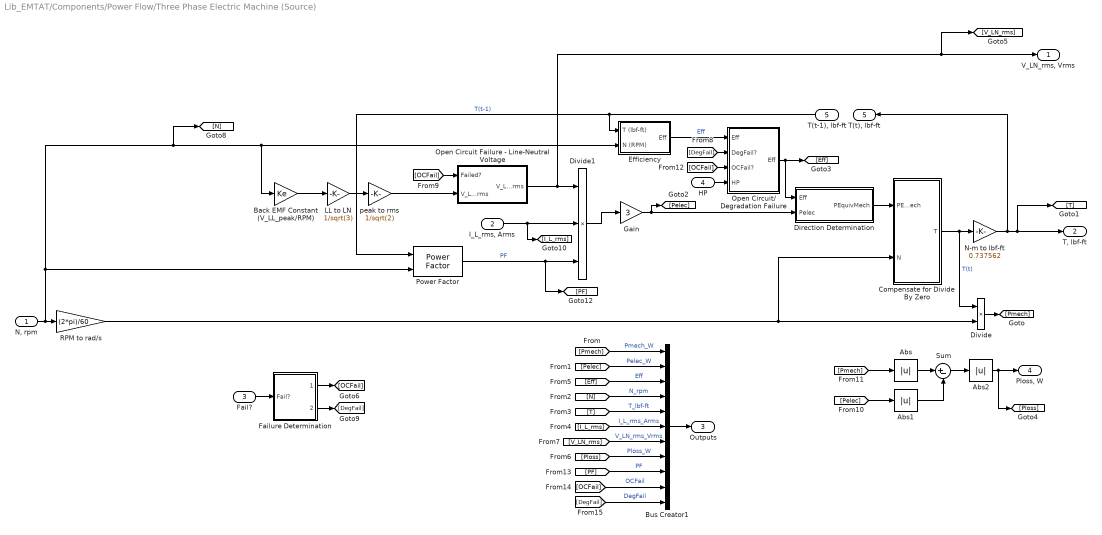
== system Lib_EMTAT/Components/Power Flow/Three Phase Electric Machine (Source) ==
  "N, rpm" : Inport
  "I_L_rms, Arms" : Inport  Port=2
  Fail? : Inport  Port=3
  HP : Inport  Port=4
  "T(t-1), lbf-ft" : Inport  Port=5
  Abs : Abs  SaturateOnIntegerOverflow=off
  Abs1 : Abs  SaturateOnIntegerOverflow=off
  Abs2 : Abs  SaturateOnIntegerOverflow=off
  Back EMF Constant (V_LL_peak/RPM) : Gain  Gain=Ke
  Bus Creator1 : BusCreator  Inputs=11
  Compensate for Divide By Zero : Subsystem
  Direction Determination : Subsystem
  Divide : Product  Inputs=**
  Divide1 : Product  Inputs=***
  Efficiency : Subsystem
  Failure Determination : Subsystem
  Gain : Gain  Gain=3
  LL to LN : Gain  Gain=1/sqrt(3)
  N-m to lbf-ft : Gain  Gain=0.737562
  Open Circuit Failure - Line-Neutral Voltage : Subsystem
  Open Circuit/ Degradation Failure : Subsystem
  Power Factor : $bdroot/Components/Power Flow/Three Phase Electric Machine (Sink)/Power Factor  SystemSampleTime=-1  VariantActivationTime=update diagram  AllowFlexibleInterface=on  Latency=0  AutoFrameSizeCalculation=off
  RPM to rad/s : Gain  Gain=(2*pi)/60
  Sum : Sum  Inputs=|+-
  peak to rms : Gain  Gain=1/sqrt(2)
  "V_LN_rms, Vrms" : Outport
  "T, lbf-ft" : Outport  Port=2
  Outputs : Outport  Port=3
  "Ploss, W" : Outport  Port=4
  "T(t), lbf-ft" : Outport  Port=5
  wires:
  [DegFail] -> Bus Creator1/11  "DegFail"
  [OCFail] -> Bus Creator1/10  "OCFail"
  peak to rms/1 -> Open Circuit Failure - Line-Neutral Voltage/2(V_LN_rms)
  Open Circuit Failure - Line-Neutral Voltage/1("V_LN_rms ") -> "V_LN_rms, Vrms"/1, [V_LN_rms], Divide1/1
  [OCFail] -> Open Circuit Failure - Line-Neutral Voltage/1(Failed?)
  Open Circuit/ Degradation Failure/1("Eff ") -> Direction Determination/1(Eff), [Eff]
  HP/1 -> Open Circuit/ Degradation Failure/4(HP)
  [DegFail] -> Open Circuit/ Degradation Failure/2(DegFail?)
  Efficiency/1(Eff) -> Open Circuit/ Degradation Failure/1(Eff)  "Eff"
  [OCFail] -> Open Circuit/ Degradation Failure/3(OCFail?)
  Failure Determination/1(OCFail) -> [OCFail]
  Failure Determination/2(DegFail) -> [DegFail]
  Fail?/1 -> Failure Determination/1(Fail?)
  N-m to lbf-ft/1 -> "T, lbf-ft"/1, [T], "T(t), lbf-ft"/1
  Gain/1 -> Direction Determination/2(Pelec), [Pelec]
  LL to LN/1 -> peak to rms/1
  [Pmech] -> Abs/1
  [Pelec] -> Abs1/1
  Divide/1 -> [Pmech]
  Abs2/1 -> "Ploss, W"/1, [Ploss]
  Sum/1 -> Abs2/1
  Abs1/1 -> Sum/2
  Abs/1 -> Sum/1
  Bus Creator1/1 -> Outputs/1
  Direction Determination/1(PEquivMech) -> Compensate for Divide By Zero/1(PEquivMech)
  "T(t-1), lbf-ft"/1 -> Power Factor/1, Efficiency/1(T (lbf-ft))  "T(t-1)"
  Compensate for Divide By Zero/1(T) -> N-m to lbf-ft/1, Divide/1  "T(t)"
  Divide1/1 -> Gain/1
  Back EMF Constant (V_LL_peak/RPM)/1 -> LL to LN/1
  [V_LN_rms] -> Bus Creator1/7  "V_LN_rms_Vrms"
  [I_L_rms] -> Bus Creator1/6  "I_L_rms_Arms"
  [Eff] -> Bus Creator1/3  "Eff"
  [T] -> Bus Creator1/5  "T_lbf-ft"
  [N] -> Bus Creator1/4  "N_rpm"
  [Pmech] -> Bus Creator1/1  "Pmech_W"
  [Ploss] -> Bus Creator1/8  "Ploss_W"
  [Pelec] -> Bus Creator1/2  "Pelec_W"
  RPM to rad/s/1 -> Compensate for Divide By Zero/2(N), Divide/2
  "I_L_rms, Arms"/1 -> Divide1/2, [I_L_rms]
  "N, rpm"/1 -> RPM to rad/s/1, Efficiency/2(N (RPM)), Back EMF Constant (V_LL_peak/RPM)/1, [N], Power Factor/2
  Power Factor/1 -> [PF], Divide1/3  "PF"
  [PF] -> Bus Creator1/9  "PF"

== system Lib_EMTAT/Components/Power Flow/AC-AC Transformer (Efficiency Map)/Compensate for Divide By Zero ==
  note: If Vin is not equal to zero, use its value.
      | If Vin is equal to zero, it will calculate a nan value for Iin. Set Iin to zero.
  P_AC_1 : Inport
  V_LN_rms_1 : Inport  Port=2
  Fix Divide By Zero. : Subsystem
  I_L_rms_1 : Outport
  wires:
  Fix Divide By Zero./1(I_L_rms_1) -> I_L_rms_1/1
  P_AC_1/1 -> Fix Divide By Zero./2(P_AC_1)
  V_LN_rms_1/1 -> Fix Divide By Zero./1(V_LN_rms_1)

== system Lib_EMTAT/Components/Power Flow/AC-AC Transformer (Efficiency Map)/Direction Determination ==
  P_AC_2 : Inport
  Eff : Inport  Port=2
  Divide : Product  Inputs=/*
  Divide1 : Product  Inputs=**
  Switch : Switch  Criteria=u2 > Threshold  SaturateOnIntegerOverflow=off  InputSameDT=off
  P_AC_1 : Outport
  wires:
  P_AC_2/1 -> Divide1/1, Divide/2, Switch/2
  Divide/1 -> Switch/1
  Divide1/1 -> Switch/3
  Eff/1 -> Divide/1, Divide1/2
  Switch/1 -> P_AC_1/1

== system Lib_EMTAT/Components/Power Flow/AC-AC Transformer (Efficiency Map)/Efficiency ==
  V_LN_rms_1 : Inport
  I_L_rms_2 : Inport  Port=2
  2-D Lookup Table : Lookup_n-D  BreakpointsForDimension1=X_C_VoltageAC1Vec_M  BreakpointsForDimension2=Y_C_CurrentAC2Vec_M  Table=T_C_EffArray_M  ExtrapMethod=Clip  UseLastTableValue=on  InternalRulePriority=Speed  RndMeth=Simplest
      settings: InputPortMap=u0,u1
  Abs : Abs  SaturateOnIntegerOverflow=off
  Abs1 : Abs  SaturateOnIntegerOverflow=off
  Eff : Outport
  wires:
  2-D Lookup Table/1 -> Eff/1
  I_L_rms_2/1 -> Abs1/1
  Abs1/1 -> 2-D Lookup Table/2
  Abs/1 -> 2-D Lookup Table/1
  V_LN_rms_1/1 -> Abs/1

== system Lib_EMTAT/Components/Power Flow/AC-AC Transformer (Efficiency Map)/Failure Determination ==
  Fail? : Inport
  Compare To Constant : simulink/Logic and Bit Operations/Compare To Constant  relop===  const=1  OutDataTypeStr=boolean
  Compare To Constant1 : simulink/Logic and Bit Operations/Compare To Constant  relop===  const=2  OutDataTypeStr=boolean
  Data Type Conversion : DataTypeConversion  OutDataTypeStr=double  SaturateOnIntegerOverflow=off  RndMeth=Floor
  Data Type Conversion1 : DataTypeConversion  OutDataTypeStr=double  SaturateOnIntegerOverflow=off  RndMeth=Floor
  Failure Mode : Constant  Value=FM
  Logical Operator : Logic  AllPortsSameDT=off  OutDataTypeStr=boolean
  Logical Operator1 : Logic  AllPortsSameDT=off  OutDataTypeStr=boolean
  OCFail : Outport
  DegFail : Outport  Port=2
  wires:
  Data Type Conversion/1 -> OCFail/1
  Data Type Conversion1/1 -> DegFail/1
  Fail?/1 -> Logical Operator/2, Logical Operator1/2
  Logical Operator1/1 -> Data Type Conversion1/1
  Compare To Constant1/1 -> Logical Operator1/1
  Logical Operator/1 -> Data Type Conversion/1
  Compare To Constant/1 -> Logical Operator/1
  Failure Mode/1 -> Compare To Constant/1, Compare To Constant1/1

== system Lib_EMTAT/Components/Power Flow/AC-AC Transformer (Efficiency Map)/Open Circuit Failure - DC Current ==
  Failed? : Inport
  I_L_rms_1 : Inport  Port=2
  Constant : Constant  Value=0
  IsInf : RelationalOperator  Operator=isInf  OutDataTypeStr=boolean  RndMeth=Simplest  InputSameDT=off
  IsNaN : RelationalOperator  Operator=isNaN  OutDataTypeStr=boolean  RndMeth=Simplest  InputSameDT=off
  Logical Operator : Logic  Operator=OR  Inputs=3  AllPortsSameDT=off  OutDataTypeStr=boolean
  Switch : Switch  Criteria=u2 > Threshold  SaturateOnIntegerOverflow=off  InputSameDT=off
  "I_L_rms_1 " : Outport
  wires:
  IsInf/1 -> Logical Operator/3
  IsNaN/1 -> Logical Operator/2
  Logical Operator/1 -> Switch/2
  Switch/1 -> "I_L_rms_1 "/1
  I_L_rms_1/1 -> Switch/3, IsInf/1, IsNaN/1
  Constant/1 -> Switch/1
  Failed?/1 -> Logical Operator/1

== system Lib_EMTAT/Components/Power Flow/AC-AC Transformer (Efficiency Map)/Open Circuit Failure - Line to Neutral Voltage ==
  Failed? : Inport
  V_LN_rms_2 : Inport  Port=2
  Constant : Constant  Value=0
  IsInf : RelationalOperator  Operator=isInf  OutDataTypeStr=boolean  RndMeth=Simplest  InputSameDT=off
  IsNaN : RelationalOperator  Operator=isNaN  OutDataTypeStr=boolean  RndMeth=Simplest  InputSameDT=off
  Logical Operator : Logic  Operator=OR  Inputs=3  AllPortsSameDT=off  OutDataTypeStr=boolean
  Switch : Switch  Criteria=u2 > Threshold  SaturateOnIntegerOverflow=off  InputSameDT=off
  "V_LN_rms_2 " : Outport
  wires:
  Failed?/1 -> Logical Operator/1
  Constant/1 -> Switch/1
  V_LN_rms_2/1 -> IsNaN/1, IsInf/1, Switch/3
  Switch/1 -> "V_LN_rms_2 "/1
  Logical Operator/1 -> Switch/2
  IsNaN/1 -> Logical Operator/2
  IsInf/1 -> Logical Operator/3

== system Lib_EMTAT/Components/Power Flow/AC-AC Transformer (Efficiency Map)/Open Circuit// Degradation Failure ==
  Eff : Inport
  DegFail? : Inport  Port=2
  OCFail? : Inport  Port=3
  HP : Inport  Port=4
  Constant : Constant  Value=eps
  Constant1 : Constant
  Divide : Product  Inputs=**
  "If degradation failure, scale Eff." : Switch  Criteria=u2 > Threshold  SaturateOnIntegerOverflow=off  InputSameDT=off
  "If open circuit failure, set Eff = eps." : Switch  Criteria=u2 > Threshold  SaturateOnIntegerOverflow=off  InputSameDT=off
  Sum : Sum  Inputs=+-|
  "Eff " : Outport
  wires:
  DegFail?/1 -> "If degradation failure, scale Eff."/2
  "If degradation failure, scale Eff."/1 -> "If open circuit failure, set Eff = eps."/3
  Divide/1 -> "If degradation failure, scale Eff."/1
  "If open circuit failure, set Eff = eps."/1 -> "Eff "/1
  OCFail?/1 -> "If open circuit failure, set Eff = eps."/2
  Constant/1 -> "If open circuit failure, set Eff = eps."/1
  Sum/1 -> Divide/1
  Eff/1 -> "If degradation failure, scale Eff."/3, Divide/2
  HP/1 -> Sum/2
  Constant1/1 -> Sum/1

== system Lib_EMTAT/Components/Power Flow/AC-AC Transformer (Power Loss Map)/Compensate for Divide By Zero ==
  note: If Vin is not equal to zero, use its value.
      | If Vin is equal to zero, it will calculate a nan value for Iin. Set Iin to zero.
  P_AC_1 : Inport
  V_LN_rms_1 : Inport  Port=2
  Fix Divide By Zero. : Subsystem
  I_L_rms_1 : Outport
  wires:
  V_LN_rms_1/1 -> Fix Divide By Zero./1(V_LN_rms_1)
  P_AC_1/1 -> Fix Divide By Zero./2(P_AC_1)
  Fix Divide By Zero./1(I_L_rms_1) -> I_L_rms_1/1

== system Lib_EMTAT/Components/Power Flow/AC-AC Transformer (Power Loss Map)/Direction Determination ==
  P_AC_2 : Inport
  Ploss : Inport  Port=2
  Add1 : Sum
  Switch : Switch  Criteria=u2 ~= 0  SaturateOnIntegerOverflow=off  InputSameDT=off
  P_AC_1 : Outport
  wires:
  Add1/1 -> Switch/1
  Switch/1 -> P_AC_1/1
  P_AC_2/1 -> Switch/2, Switch/3, Add1/2
  Ploss/1 -> Add1/1

== system Lib_EMTAT/Components/Power Flow/AC-AC Transformer (Power Loss Map)/Efficiency ==
  P_AC_2 : Inport
  P_AC_1 : Inport  Port=2
  Abs : Abs  SaturateOnIntegerOverflow=off
  Abs1 : Abs  SaturateOnIntegerOverflow=off
  Fix Divide By Zero. : Subsystem
  Fix Divide By Zero.1 : Subsystem
  GreaterThan : RelationalOperator  OutDataTypeStr=boolean  RndMeth=Simplest  InputSameDT=off
  Switch : Switch  Criteria=u2 > Threshold  SaturateOnIntegerOverflow=off  InputSameDT=off
  Eff : Outport
  wires:
  Switch/1 -> Eff/1
  GreaterThan/1 -> Switch/2
  Abs1/1 -> Fix Divide By Zero.1/2(abs(P_AC_2)), Fix Divide By Zero./1(abs(P_AC_2)), GreaterThan/2
  P_AC_1/1 -> Abs/1
  P_AC_2/1 -> Abs1/1
  Abs/1 -> Fix Divide By Zero.1/1(abs(P_AC_1)), Fix Divide By Zero./2(abs(P_AC_1)), GreaterThan/1
  Fix Divide By Zero./1(Eff) -> Switch/3
  Fix Divide By Zero.1/1(Eff) -> Switch/1

== system Lib_EMTAT/Components/Power Flow/AC-AC Transformer (Power Loss Map)/Failure Determination ==
  Fail? : Inport
  Compare To Constant : simulink/Logic and Bit Operations/Compare To Constant  relop===  const=1  OutDataTypeStr=boolean
  Compare To Constant1 : simulink/Logic and Bit Operations/Compare To Constant  relop===  const=2  OutDataTypeStr=boolean
  Data Type Conversion : DataTypeConversion  OutDataTypeStr=double  SaturateOnIntegerOverflow=off  RndMeth=Floor
  Data Type Conversion1 : DataTypeConversion  OutDataTypeStr=double  SaturateOnIntegerOverflow=off  RndMeth=Floor
  Failure Mode : Constant  Value=FM
  Logical Operator : Logic  AllPortsSameDT=off  OutDataTypeStr=boolean
  Logical Operator1 : Logic  AllPortsSameDT=off  OutDataTypeStr=boolean
  OCFail : Outport
  DegFail : Outport  Port=2
  wires:
  Failure Mode/1 -> Compare To Constant1/1, Compare To Constant/1
  Compare To Constant/1 -> Logical Operator/1
  Logical Operator/1 -> Data Type Conversion/1
  Compare To Constant1/1 -> Logical Operator1/1
  Logical Operator1/1 -> Data Type Conversion1/1
  Fail?/1 -> Logical Operator1/2, Logical Operator/2
  Data Type Conversion1/1 -> DegFail/1
  Data Type Conversion/1 -> OCFail/1

== system Lib_EMTAT/Components/Power Flow/AC-AC Transformer (Power Loss Map)/Open Circuit Failure - DC Current ==
  Failed? : Inport
  I_L_rms_1 : Inport  Port=2
  Constant : Constant  Value=0
  IsInf : RelationalOperator  Operator=isInf  OutDataTypeStr=boolean  RndMeth=Simplest  InputSameDT=off
  IsNaN : RelationalOperator  Operator=isNaN  OutDataTypeStr=boolean  RndMeth=Simplest  InputSameDT=off
  Logical Operator : Logic  Operator=OR  Inputs=3  AllPortsSameDT=off  OutDataTypeStr=boolean
  Switch : Switch  Criteria=u2 > Threshold  SaturateOnIntegerOverflow=off  InputSameDT=off
  "I_L_rms_1 " : Outport
  wires:
  Failed?/1 -> Logical Operator/1
  Constant/1 -> Switch/1
  I_L_rms_1/1 -> IsNaN/1, IsInf/1, Switch/3
  Switch/1 -> "I_L_rms_1 "/1
  Logical Operator/1 -> Switch/2
  IsNaN/1 -> Logical Operator/2
  IsInf/1 -> Logical Operator/3

== system Lib_EMTAT/Components/Power Flow/AC-AC Transformer (Power Loss Map)/Open Circuit Failure - Line to Neutral Voltage ==
  Failed? : Inport
  V_LN_rms_2 : Inport  Port=2
  Constant : Constant  Value=0
  IsInf : RelationalOperator  Operator=isInf  OutDataTypeStr=boolean  RndMeth=Simplest  InputSameDT=off
  IsNaN : RelationalOperator  Operator=isNaN  OutDataTypeStr=boolean  RndMeth=Simplest  InputSameDT=off
  Logical Operator : Logic  Operator=OR  Inputs=3  AllPortsSameDT=off  OutDataTypeStr=boolean
  Switch : Switch  Criteria=u2 > Threshold  SaturateOnIntegerOverflow=off  InputSameDT=off
  "V_LN_rms_2 " : Outport
  wires:
  IsInf/1 -> Logical Operator/3
  IsNaN/1 -> Logical Operator/2
  Logical Operator/1 -> Switch/2
  Switch/1 -> "V_LN_rms_2 "/1
  V_LN_rms_2/1 -> Switch/3, IsInf/1, IsNaN/1
  Constant/1 -> Switch/1
  Failed?/1 -> Logical Operator/1

== system Lib_EMTAT/Components/Power Flow/AC-AC Transformer (Power Loss Map)/Open Circuit// Degradation Failure ==
  Ploss : Inport
  DegFail? : Inport  Port=2
  OCFail? : Inport  Port=3
  HP : Inport  Port=4
  Constant : Constant  Value=0
  Constant1 : Constant  Value=Plosslim
  Divide : Product  Inputs=**
  "If degradation failure, add to Ploss." : Switch  Criteria=u2 > Threshold  SaturateOnIntegerOverflow=off  InputSameDT=off
  "If open circuit failure, set Ploss = 0." : Switch  Criteria=u2 > Threshold  SaturateOnIntegerOverflow=off  InputSameDT=off
  Sum1 : Sum  Inputs=++|
  "Ploss " : Outport
  wires:
  DegFail?/1 -> "If degradation failure, add to Ploss."/2
  "If degradation failure, add to Ploss."/1 -> "If open circuit failure, set Ploss = 0."/3
  Ploss/1 -> Sum1/2, "If degradation failure, add to Ploss."/3
  Sum1/1 -> "If degradation failure, add to Ploss."/1
  HP/1 -> Divide/2
  "If open circuit failure, set Ploss = 0."/1 -> "Ploss "/1
  OCFail?/1 -> "If open circuit failure, set Ploss = 0."/2
  Constant/1 -> "If open circuit failure, set Ploss = 0."/1
  Constant1/1 -> Divide/1
  Divide/1 -> Sum1/1

== system Lib_EMTAT/Components/Power Flow/AC-AC Transformer (Power Loss Map)/Power Loss ==
  V_LN_rms_1 : Inport
  I_L_rms_2 : Inport  Port=2
  2-D Lookup Table : Lookup_n-D  BreakpointsForDimension1=X_C_VoltageAC1Vec_M  BreakpointsForDimension2=Y_C_CurrentAC2Vec_M  Table=T_C_PowLossArray_M  ExtrapMethod=Clip  UseLastTableValue=on  InternalRulePriority=Speed  RndMeth=Simplest
      settings: InputPortMap=u0,u1
  Abs : Abs  SaturateOnIntegerOverflow=off
  Abs1 : Abs  SaturateOnIntegerOverflow=off
  Saturation : Saturate  UpperLimit=inf  LowerLimit=0
  Ploss : Outport
  wires:
  V_LN_rms_1/1 -> Abs/1
  Abs/1 -> 2-D Lookup Table/1
  Abs1/1 -> 2-D Lookup Table/2
  I_L_rms_2/1 -> Abs1/1
  2-D Lookup Table/1 -> Saturation/1
  Saturation/1 -> Ploss/1

== system Lib_EMTAT/Components/Power Flow/AC-DC Rectifier (Efficiency Map)/Compensate for Divide By Zero. ==
  note: If Vin is not equal to zero, use its value.
      | If Vin is equal to zero, it will calculate a nan value for Iin. Set Iin to zero.
  PEquivAC : Inport
  V_LN_rms : Inport  Port=2
  PF : Inport  Port=3
  Constant1 : Constant  Value=eps
  Divide1 : Product  Inputs=/*
  Divide2 : Product  Inputs=**
  Switch1 : Switch  Criteria=u2 ~= 0  SaturateOnIntegerOverflow=off  InputSameDT=off
  I_L_rms : Outport
  wires:
  Divide1/1 -> I_L_rms/1
  PEquivAC/1 -> Divide1/2
  Constant1/1 -> Switch1/3
  Divide2/1 -> Switch1/2, Switch1/1
  Switch1/1 -> Divide1/1
  V_LN_rms/1 -> Divide2/2
  PF/1 -> Divide2/1

== system Lib_EMTAT/Components/Power Flow/AC-DC Rectifier (Efficiency Map)/Direction Determination ==
  P_DC : Inport
  Eff : Inport  Port=2
  Divide : Product  Inputs=**
  Divide1 : Product  Inputs=*/
  Switch : Switch  Criteria=u2 > Threshold  SaturateOnIntegerOverflow=off  InputSameDT=off
  PEquivAC : Outport
  wires:
  P_DC/1 -> Divide1/1, Divide/2, Switch/2
  Divide/1 -> Switch/1
  Divide1/1 -> Switch/3
  Eff/1 -> Divide/1, Divide1/2
  Switch/1 -> PEquivAC/1

== system Lib_EMTAT/Components/Power Flow/AC-DC Rectifier (Efficiency Map)/Efficiency ==
  V_DC : Inport
  I_L_rms : Inport  Port=2
  2-D Lookup Table : Lookup_n-D  BreakpointsForDimension1=X_C_VoltageInVec_M  BreakpointsForDimension2=Y_C_RMSCurrentOutVec_M  Table=T_C_EffArray_M  ExtrapMethod=Clip  UseLastTableValue=on  InternalRulePriority=Speed  RndMeth=Simplest
      settings: InputPortMap=u0,u1
  Abs : Abs  SaturateOnIntegerOverflow=off
  Abs1 : Abs  SaturateOnIntegerOverflow=off
  Eff : Outport
  wires:
  2-D Lookup Table/1 -> Eff/1
  I_L_rms/1 -> Abs1/1
  Abs1/1 -> 2-D Lookup Table/2
  Abs/1 -> 2-D Lookup Table/1
  V_DC/1 -> Abs/1

== system Lib_EMTAT/Components/Power Flow/AC-DC Rectifier (Efficiency Map)/Failure Determination ==
  Fail? : Inport
  Compare To Constant : simulink/Logic and Bit Operations/Compare To Constant  relop===  const=1  OutDataTypeStr=boolean
  Compare To Constant1 : simulink/Logic and Bit Operations/Compare To Constant  relop===  const=2  OutDataTypeStr=boolean
  Data Type Conversion : DataTypeConversion  OutDataTypeStr=double  SaturateOnIntegerOverflow=off  RndMeth=Floor
  Data Type Conversion1 : DataTypeConversion  OutDataTypeStr=double  SaturateOnIntegerOverflow=off  RndMeth=Floor
  Failure Mode : Constant  Value=FM
  Logical Operator : Logic  AllPortsSameDT=off  OutDataTypeStr=boolean
  Logical Operator1 : Logic  AllPortsSameDT=off  OutDataTypeStr=boolean
  OCFail : Outport
  DegFail : Outport  Port=2
  wires:
  Data Type Conversion/1 -> OCFail/1
  Data Type Conversion1/1 -> DegFail/1
  Fail?/1 -> Logical Operator/2, Logical Operator1/2
  Logical Operator1/1 -> Data Type Conversion1/1
  Compare To Constant1/1 -> Logical Operator1/1
  Logical Operator/1 -> Data Type Conversion/1
  Compare To Constant/1 -> Logical Operator/1
  Failure Mode/1 -> Compare To Constant/1, Compare To Constant1/1
